simulink model "complex_multiply_example"  (R2023a)
settings: Solver=FixedStepDiscrete  StartTime=0.0  StopTime=100  RelTol=1e-3
PostLoadFcn:
  | % Default delay values
  | D1 = 1;
  | D2 = 1;
  | D3 = 1;
  | D4 = 1;
  | D5 = 1;
InitFcn:
  | % Complex mult input DT
  | InputWL = 18;
  | InputFL = 17;
  | 
  | % Full-precision mult DT
  | MultWL = InputWL*2+1;
  | MultFL = InputFL*2;
  | IntBits = MultWL - MultFL; % integer bits
  | 
  | % Mult DT after rounding
  | OutputWL = 18;
  | OutputFL = OutputWL - IntBits;
settings Model: DataTypeOverride=Off  Creator=cchung  LastModifiedBy=cchung
settings SolverCC: AlgebraicLoopSolver=TrustRegion
settings DataIOCC: LimitDataPoints=on  SaveFormat=Array  SaveOutput=off  SaveTime=off  ReturnWorkspaceOutputs=off
settings OptimizationCC: BlockReduction=off  BooleanDataType=off  ConditionallyExecuteInputs=off  DefaultParameterBehavior=Inlined  LifeSpan=inf
settings DebuggingCC: AlgebraicLoopMsg=error  SaveWithParameterizedLinksMsg=none  UnderspecifiedInitializationDetection=Classic  MergeDetectMultiDrivingBlocksExec=none  SignalResolutionControl=TryResolveAllWithWarning  SingleTaskRateTransMsg=error  UnconnectedInputMsg=warning  UnconnectedOutputMsg=warning  UnconnectedLineMsg=warning  StrictBusMsg=ErrorOnBusTreatedAsVector  SFUnexpectedBacktrackingDiag=warning  SFNoUnconditionalDefaultTransitionDiag=warning  SFExecutionAtInitializationDiag=none  ArithmeticOperatorsInVariantConditions=warning
settings HardwareCC: ProdBitPerPointer=32  ProdBitPerSizeT=32  ProdBitPerPtrDiffT=32  ProdLargestAtomicFloat=None  ProdIntDivRoundTo=Undefined  ProdEndianess=Unspecified  ProdWordSize=32  ProdHWDeviceType=ASIC/FPGA->ASIC/FPGA  TargetUnknown=on  ProdEqTarget=off
settings ModelReferenceCC: EnableRefExpFcnMdlSchedulingChecks=on  PropagateSignalLabelsOutOfModel=off
settings SFSimCC: SimUseLocalCustomCode=off  CustomCodeUndefinedFunction=UseInterfaceOnly
settings RTWCC: RTWUseLocalCustomCode=off
settings CodeAppCC: StateflowObjectComments=on
settings GRTTargetCC: TargetLangStandard=C89/C90 (ANSI)
settings ConfigComp: CovMetricSettings=dw  CovSaveCumulativeToWorkspaceVar=on  CovSaveSingleToWorkspaceVar=on  CovExternalEMLEnable=off

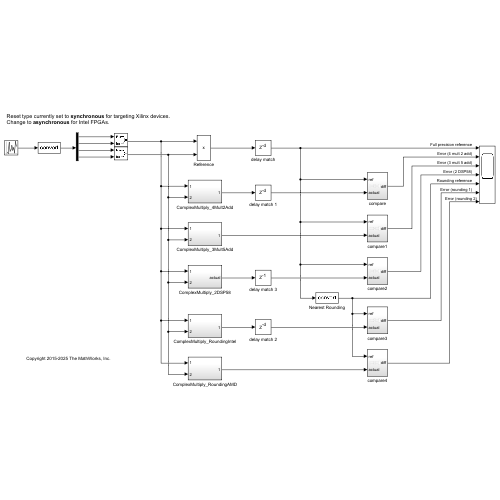
[thumbnail: Simulink's stored preview of the top-level diagram]
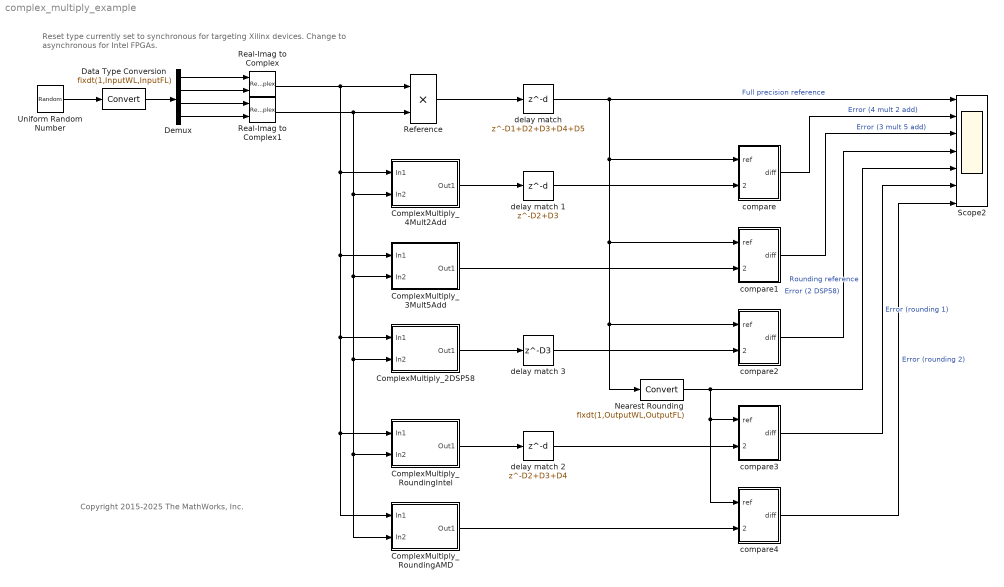
== system complex_multiply_example ==
  note: Copyright 2015-2025 The MathWorks, Inc.
  note: Reset type currently set to synchronous for targeting Xilinx devices.
      | Change to asynchronous for Intel FPGAs.
  ComplexMultiply_2DSP58 : Subsystem
  ComplexMultiply_3Mult5Add : Subsystem
  ComplexMultiply_4Mult2Add : Subsystem
  ComplexMultiply_RoundingAMD : Subsystem
  ComplexMultiply_RoundingIntel : Subsystem
  Data Type Conversion : DataTypeConversion  OutDataTypeStr=fixdt(1,InputWL,InputFL)  RndMeth=Floor
  Demux : Demux
  Nearest Rounding : DataTypeConversion  OutDataTypeStr=fixdt(1,OutputWL,OutputFL)  RndMeth=Nearest  SaturateOnIntegerOverflow=off
  Real-Imag to Complex : RealImagToComplex
  Real-Imag to Complex1 : RealImagToComplex
  Reference : Product  OutDataTypeStr=fixdt(1,MultWL,MultFL)
  Scope2 : Scope  NumInputPorts=7
  Uniform Random Number : UniformRandomNumber  Minimum=-1*ones(1,4)  Maximum=ones(1,4)  Seed=randi([0 100],1,4)  SampleTime=1
  compare : Subsystem
  compare1 : Subsystem
  compare2 : Subsystem
  compare3 : Subsystem
  compare4 : Subsystem
  delay match : Delay  DelayLength=D1+D2+D3+D4+D5
  delay match 1 : Delay  DelayLength=D2+D3
  delay match 2 : Delay  DelayLength=D2+D3+D4
  delay match 3 : Delay  DelayLength=D3
  wires:
  ComplexMultiply_4Mult2Add/1(Out1) -> delay match 1/1
  Real-Imag to Complex/1 -> ComplexMultiply_2DSP58/1(In1), ComplexMultiply_RoundingAMD/1(In1), ComplexMultiply_RoundingIntel/1(In1), ComplexMultiply_3Mult5Add/1(In1), ComplexMultiply_4Mult2Add/1(In1), Reference/1
  Real-Imag to Complex1/1 -> ComplexMultiply_3Mult5Add/2(In2), ComplexMultiply_2DSP58/2(In2), ComplexMultiply_RoundingAMD/2(In2), ComplexMultiply_RoundingIntel/2(In2), ComplexMultiply_4Mult2Add/2(In2), Reference/2
  Reference/1 -> delay match/1
  delay match 1/1 -> compare/2(actual)
  ComplexMultiply_3Mult5Add/1(Out1) -> compare1/2(actual)
  Uniform Random Number/1 -> Data Type Conversion/1
  Data Type Conversion/1 -> Demux/1
  Demux/1 -> Real-Imag to Complex/1
  ComplexMultiply_RoundingIntel/1(Out1) -> delay match 2/1
  delay match/1 -> compare2/1(ref), Nearest Rounding/1, compare1/1(ref), compare/1(ref), Scope2/1  "Full precision reference"
  compare/1(diff) -> Scope2/2  "Error (4 mult 2 add)"
  compare1/1(diff) -> Scope2/3  "Error (3 mult 5 add)"
  delay match 2/1 -> compare3/2(actual)
  Nearest Rounding/1 -> compare4/1(ref), compare3/1(ref), Scope2/5  "Rounding reference"
  Demux/2 -> Real-Imag to Complex/2
  Demux/3 -> Real-Imag to Complex1/1
  Demux/4 -> Real-Imag to Complex1/2
  compare3/1(diff) -> Scope2/6  "Error (rounding 1)"
  ComplexMultiply_RoundingAMD/1(Out1) -> compare4/2(actual)
  compare4/1(diff) -> Scope2/7  "Error (rounding 2)"
  ComplexMultiply_2DSP58/1(Out1) -> delay match 3/1
  delay match 3/1 -> compare2/2(actual)
  compare2/1(diff) -> Scope2/4  "Error (2 DSP58)"

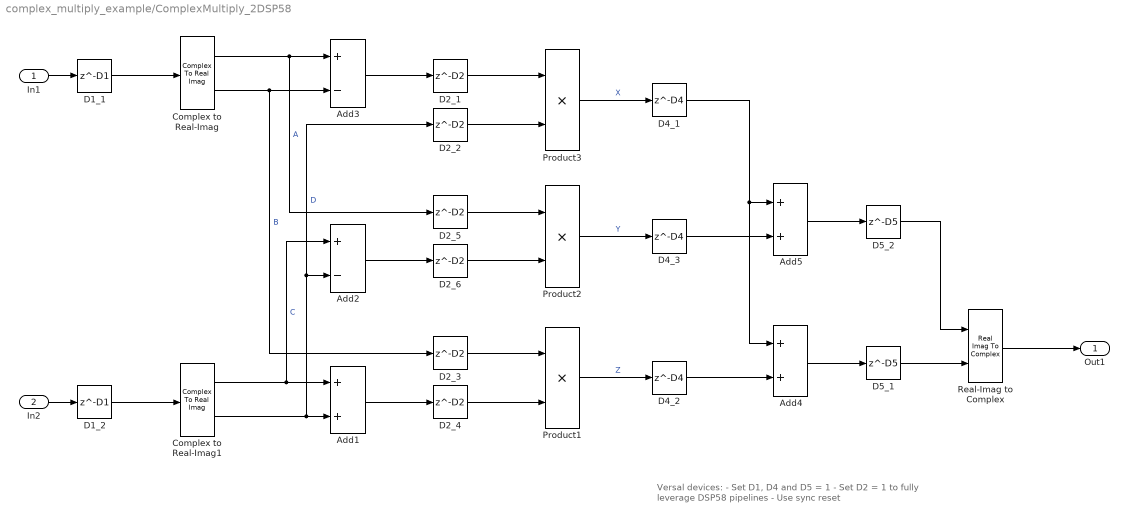
== system complex_multiply_example/ComplexMultiply_2DSP58 ==
  note: Versal devices:
      | - Set D1, D4 and D5 = 1
      | - Set D2 = 1 to fully leverage DSP58 pipelines
      | - Use sync reset
  In1 : Inport
  In2 : Inport  Port=2
  Add1 : Sum
  Add2 : Sum  Inputs=+-
  Add3 : Sum  Inputs=+-
  Add4 : Sum
  Add5 : Sum
  Complex to Real-Imag : ComplexToRealImag
  Complex to Real-Imag1 : ComplexToRealImag
  D1_1 : Delay  DelayLength=D1
  D1_2 : Delay  DelayLength=D1
  D2_{1..6} (6 alike) : Delay  DelayLength=D2
  D4_1 : Delay  DelayLength=D4
  D4_2 : Delay  DelayLength=D4
  D4_3 : Delay  DelayLength=D4
  D5_1 : Delay  DelayLength=D5
  D5_2 : Delay  DelayLength=D5
  Product1 : Product
  Product2 : Product
  Product3 : Product
  Real-Imag to Complex : RealImagToComplex
  Out1 : Outport  VectorParamsAs1DForOutWhenUnconnected=off
  wires:
  Real-Imag to Complex/1 -> Out1/1
  In2/1 -> D1_2/1
  Complex to Real-Imag1/1 -> Add2/1, Add1/1  "C"
  Add4/1 -> D5_1/1
  Add5/1 -> D5_2/1
  In1/1 -> D1_1/1
  D1_1/1 -> Complex to Real-Imag/1
  D1_2/1 -> Complex to Real-Imag1/1
  Complex to Real-Imag/1 -> Add3/1, D2_5/1  "A"
  Complex to Real-Imag/2 -> Add3/2, D2_3/1  "B"
  Add3/1 -> D2_1/1
  Complex to Real-Imag1/2 -> D2_2/1, Add2/2, Add1/2  "D"
  Add1/1 -> D2_4/1
  Add2/1 -> D2_6/1
  Product3/1 -> D4_1/1  "X"
  Product1/1 -> D4_2/1  "Z"
  Product2/1 -> D4_3/1  "Y"
  D5_1/1 -> Real-Imag to Complex/2
  D5_2/1 -> Real-Imag to Complex/1
  D4_1/1 -> Add4/1, Add5/1
  D4_2/1 -> Add4/2
  D4_3/1 -> Add5/2
  D2_1/1 -> Product3/1
  D2_2/1 -> Product3/2
  D2_3/1 -> Product1/1
  D2_4/1 -> Product1/2
  D2_5/1 -> Product2/1
  D2_6/1 -> Product2/2

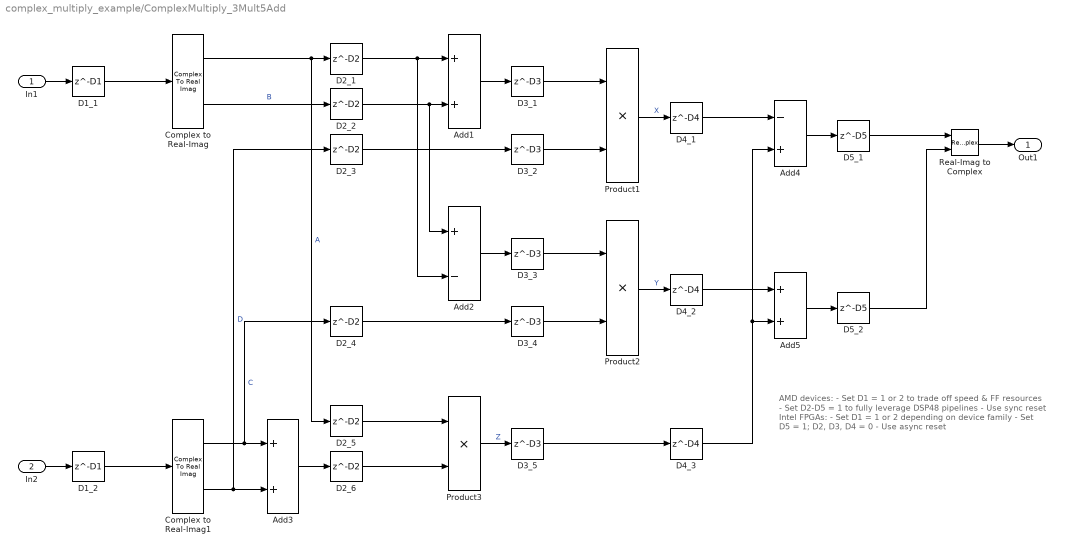
== system complex_multiply_example/ComplexMultiply_3Mult5Add ==
  note: AMD devices:
      | - Set D1 = 1 or 2 to trade off speed & FF resources
      | - Set D2-D5 = 1 to fully leverage DSP48 pipelines
      | - Use sync reset
      |
      | Intel FPGAs:
      | - Set D1 = 1 or 2 depending on device family
      | - Set D5 = 1; D2, D3, D4 = 0
      | - Use async reset
  In1 : Inport
  In2 : Inport  Port=2
  Add1 : Sum
  Add2 : Sum  Inputs=+-
  Add3 : Sum
  Add4 : Sum  Inputs=-+
  Add5 : Sum
  Complex to Real-Imag : ComplexToRealImag
  Complex to Real-Imag1 : ComplexToRealImag
  D1_1 : Delay  DelayLength=D1
  D1_2 : Delay  DelayLength=D1
  D2_{1..6} (6 alike) : Delay  DelayLength=D2
  D3_{1..5} (5 alike) : Delay  DelayLength=D3
  D4_1 : Delay  DelayLength=D4
  D4_2 : Delay  DelayLength=D4
  D4_3 : Delay  DelayLength=D4
  D5_1 : Delay  DelayLength=D5
  D5_2 : Delay  DelayLength=D5
  Product1 : Product
  Product2 : Product
  Product3 : Product
  Real-Imag to Complex : RealImagToComplex
  Out1 : Outport  VectorParamsAs1DForOutWhenUnconnected=off
  wires:
  Real-Imag to Complex/1 -> Out1/1
  In2/1 -> D1_2/1
  Complex to Real-Imag1/1 -> Add3/1, D2_4/1  "C"
  Complex to Real-Imag1/2 -> Add3/2, D2_3/1  "D"
  Product1/1 -> D4_1/1  "X"
  Product2/1 -> D4_2/1  "Y"
  Product3/1 -> D3_5/1  "Z"
  Add4/1 -> D5_1/1
  Add5/1 -> D5_2/1
  D5_1/1 -> Real-Imag to Complex/1
  D5_2/1 -> Real-Imag to Complex/2
  D4_1/1 -> Add4/1
  D4_2/1 -> Add5/1
  D3_5/1 -> D4_3/1
  Add1/1 -> D3_1/1
  Add3/1 -> D2_6/1
  Add2/1 -> D3_3/1
  Complex to Real-Imag/1 -> D2_5/1, D2_1/1  "A"
  Complex to Real-Imag/2 -> D2_2/1  "B"
  D3_1/1 -> Product1/1
  D2_6/1 -> Product3/2
  D3_3/1 -> Product2/1
  D4_3/1 -> Add4/2, Add5/2
  D3_4/1 -> Product2/2
  D3_2/1 -> Product1/2
  D2_4/1 -> D3_4/1
  D2_3/1 -> D3_2/1
  D2_5/1 -> Product3/1
  D2_2/1 -> Add1/2, Add2/1
  D2_1/1 -> Add2/2, Add1/1
  In1/1 -> D1_1/1
  D1_1/1 -> Complex to Real-Imag/1
  D1_2/1 -> Complex to Real-Imag1/1

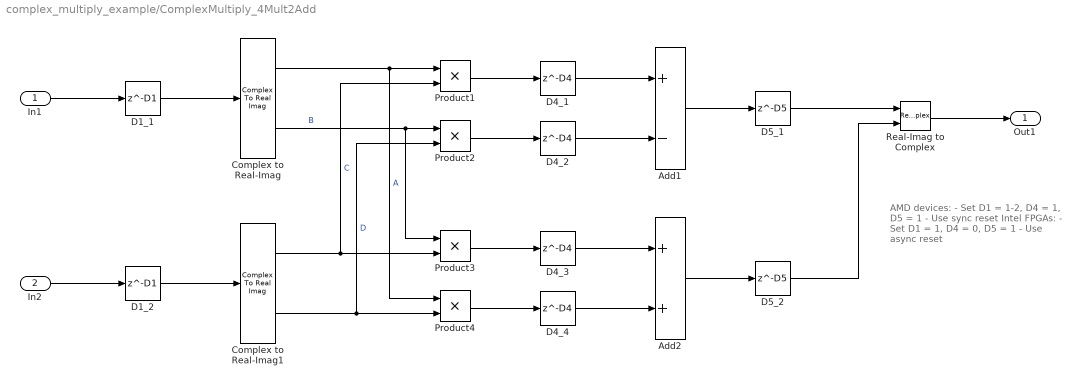
== system complex_multiply_example/ComplexMultiply_4Mult2Add ==
  note: AMD devices:
      | - Set D1 = 1-2, D4 = 1, D5 = 1
      | - Use sync reset
      |
      | Intel FPGAs:
      | - Set D1 = 1, D4 = 0, D5 = 1
      | - Use async reset
  In1 : Inport
  In2 : Inport  Port=2
  Add1 : Sum  Inputs=+-
  Add2 : Sum
  Complex to Real-Imag : ComplexToRealImag
  Complex to Real-Imag1 : ComplexToRealImag
  D1_1 : Delay  DelayLength=D1
  D1_2 : Delay  DelayLength=D1
  D4_{1..4} (4 alike) : Delay  DelayLength=D4
  D5_1 : Delay  DelayLength=D5
  D5_2 : Delay  DelayLength=D5
  Product{1..4} (4 alike) : Product
  Real-Imag to Complex : RealImagToComplex
  Out1 : Outport  VectorParamsAs1DForOutWhenUnconnected=off
  wires:
  In2/1 -> D1_2/1
  In1/1 -> D1_1/1
  Real-Imag to Complex/1 -> Out1/1
  D1_1/1 -> Complex to Real-Imag/1
  D1_2/1 -> Complex to Real-Imag1/1
  Complex to Real-Imag/1 -> Product4/1, Product1/1  "A"
  Complex to Real-Imag1/1 -> Product3/2, Product1/2  "C"
  Complex to Real-Imag/2 -> Product3/1, Product2/1  "B"
  Complex to Real-Imag1/2 -> Product4/2, Product2/2  "D"
  Product1/1 -> D4_1/1
  Product3/1 -> D4_3/1
  Add1/1 -> D5_1/1
  Add2/1 -> D5_2/1
  D5_1/1 -> Real-Imag to Complex/1
  D5_2/1 -> Real-Imag to Complex/2
  D4_1/1 -> Add1/1
  Product2/1 -> D4_2/1
  D4_3/1 -> Add2/1
  Product4/1 -> D4_4/1
  D4_2/1 -> Add1/2
  D4_4/1 -> Add2/2

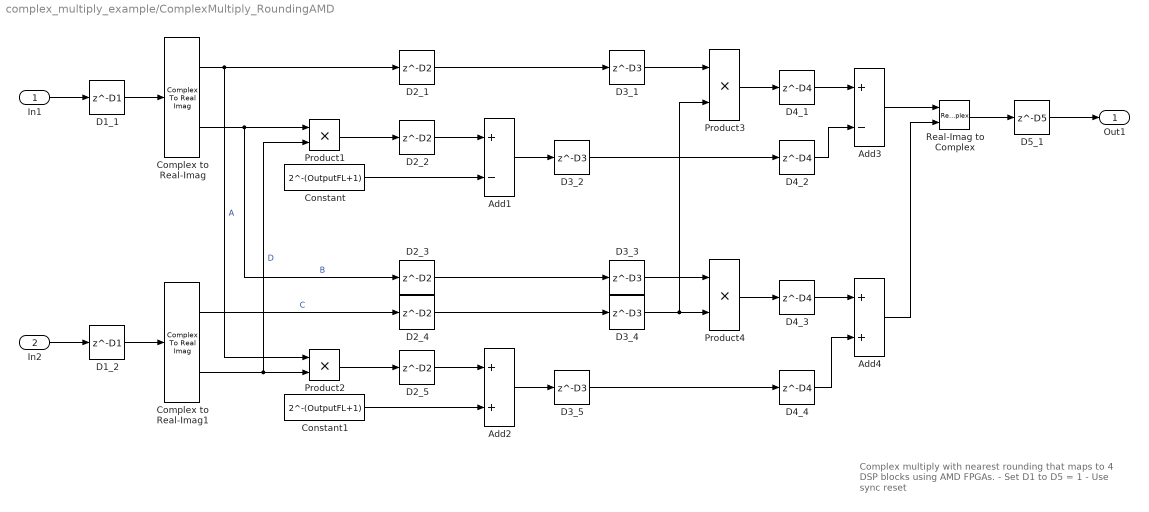
== system complex_multiply_example/ComplexMultiply_RoundingAMD ==
  note: Complex multiply with nearest rounding that maps to 4 DSP blocks using AMD FPGAs.
      |
      | - Set D1 to D5 = 1
      | - Use sync reset
  In1 : Inport
  In2 : Inport  Port=2
  Add1 : Sum  Inputs=+-
  Add2 : Sum
  Add3 : Sum  Inputs=+-  OutDataTypeStr=fixdt(1,OutputWL,OutputFL)
  Add4 : Sum  OutDataTypeStr=fixdt(1,OutputWL,OutputFL)
  Complex to Real-Imag : ComplexToRealImag
  Complex to Real-Imag1 : ComplexToRealImag
  Constant : Constant  Value=2^-(OutputFL+1)  OutDataTypeStr=Inherit: Inherit via back propagation  SampleTime=-1
  Constant1 : Constant  Value=2^-(OutputFL+1)  OutDataTypeStr=Inherit: Inherit via back propagation  SampleTime=-1
  D1_1 : Delay  DelayLength=D1
  D1_2 : Delay  DelayLength=D1
  D2_{1..5} (5 alike) : Delay  DelayLength=D2
  D3_{1..5} (5 alike) : Delay  DelayLength=D3
  D4_{1..4} (4 alike) : Delay  DelayLength=D4
  D5_1 : Delay  DelayLength=D5
  Product{1..4} (4 alike) : Product
  Real-Imag to Complex : RealImagToComplex
  Out1 : Outport  VectorParamsAs1DForOutWhenUnconnected=off
  wires:
  In2/1 -> D1_2/1
  In1/1 -> D1_1/1
  D1_1/1 -> Complex to Real-Imag/1
  D1_2/1 -> Complex to Real-Imag1/1
  Complex to Real-Imag/1 -> D2_1/1, Product2/1  "A"
  Complex to Real-Imag1/1 -> D2_4/1  "C"
  Complex to Real-Imag/2 -> Product1/1, D2_3/1  "B"
  Complex to Real-Imag1/2 -> Product2/2, Product1/2  "D"
  Product1/1 -> D2_2/1
  Real-Imag to Complex/1 -> D5_1/1
  Add1/1 -> D3_2/1
  Add4/1 -> Real-Imag to Complex/2
  D5_1/1 -> Out1/1
  Add3/1 -> Real-Imag to Complex/1
  Constant/1 -> Add1/2
  Product3/1 -> D4_1/1
  Product2/1 -> D2_5/1
  Constant1/1 -> Add2/2
  Add2/1 -> D3_5/1
  Product4/1 -> D4_3/1
  D3_5/1 -> D4_4/1
  D3_1/1 -> Product3/1
  D3_2/1 -> D4_2/1
  D3_3/1 -> Product4/1
  D3_4/1 -> Product3/2, Product4/2
  D4_1/1 -> Add3/1
  D4_2/1 -> Add3/2
  D4_3/1 -> Add4/1
  D4_4/1 -> Add4/2
  D2_1/1 -> D3_1/1
  D2_2/1 -> Add1/1
  D2_3/1 -> D3_3/1
  D2_4/1 -> D3_4/1
  D2_5/1 -> Add2/1

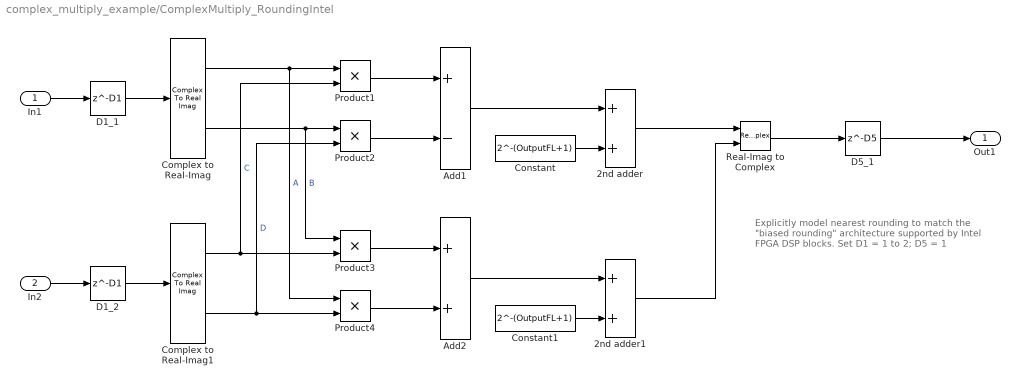
== system complex_multiply_example/ComplexMultiply_RoundingIntel ==
  note: Explicitly model nearest rounding to match the "biased rounding" architecture supported by Intel FPGA DSP blocks.
      |
      | Set D1 = 1 to 2; D5 = 1
  In1 : Inport
  In2 : Inport  Port=2
  2nd adder : Sum  OutDataTypeStr=fixdt(1,OutputWL,OutputFL)
  2nd adder1 : Sum  OutDataTypeStr=fixdt(1,OutputWL,OutputFL)
  Add1 : Sum  Inputs=+-
  Add2 : Sum
  Complex to Real-Imag : ComplexToRealImag
  Complex to Real-Imag1 : ComplexToRealImag
  Constant : Constant  Value=2^-(OutputFL+1)  OutDataTypeStr=Inherit: Inherit via back propagation  SampleTime=-1
  Constant1 : Constant  Value=2^-(OutputFL+1)  OutDataTypeStr=Inherit: Inherit via back propagation  SampleTime=-1
  D1_1 : Delay  DelayLength=D1
      settings: AttributesFormatString=ResetType : none
  D1_2 : Delay  DelayLength=D1
      settings: AttributesFormatString=ResetType : none
  D5_1 : Delay  DelayLength=D5
      settings: AttributesFormatString=ResetType : none
  Product{1..4} (4 alike) : Product
  Real-Imag to Complex : RealImagToComplex
  Out1 : Outport  VectorParamsAs1DForOutWhenUnconnected=off
  wires:
  In2/1 -> D1_2/1
  In1/1 -> D1_1/1
  D1_1/1 -> Complex to Real-Imag/1
  D1_2/1 -> Complex to Real-Imag1/1
  Complex to Real-Imag/1 -> Product4/1, Product1/1  "A"
  Complex to Real-Imag1/1 -> Product3/2, Product1/2  "C"
  Complex to Real-Imag/2 -> Product3/1, Product2/1  "B"
  Complex to Real-Imag1/2 -> Product4/2, Product2/2  "D"
  Product1/1 -> Add1/1
  Product3/1 -> Add2/1
  Product2/1 -> Add1/2
  Product4/1 -> Add2/2
  Real-Imag to Complex/1 -> D5_1/1
  Add1/1 -> 2nd adder/1
  2nd adder1/1 -> Real-Imag to Complex/2
  Add2/1 -> 2nd adder1/1
  D5_1/1 -> Out1/1
  Constant/1 -> 2nd adder/2
  Constant1/1 -> 2nd adder1/2
  2nd adder/1 -> Real-Imag to Complex/1

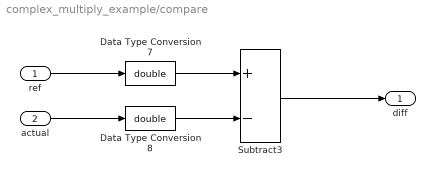
== system complex_multiply_example/compare ==
  ref : Inport
  actual : Inport  Port=2
  Data Type Conversion7 : DataTypeConversion  OutDataTypeStr=double  SaturateOnIntegerOverflow=off  RndMeth=Floor
  Data Type Conversion8 : DataTypeConversion  OutDataTypeStr=double  SaturateOnIntegerOverflow=off  RndMeth=Floor
  Subtract3 : Sum  Inputs=+-
  diff : Outport  VectorParamsAs1DForOutWhenUnconnected=off
  wires:
  actual/1 -> Data Type Conversion8/1
  Data Type Conversion7/1 -> Subtract3/1
  Data Type Conversion8/1 -> Subtract3/2
  ref/1 -> Data Type Conversion7/1
  Subtract3/1 -> diff/1

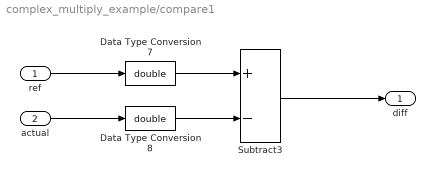
== system complex_multiply_example/compare1 ==
  ref : Inport
  actual : Inport  Port=2
  Data Type Conversion7 : DataTypeConversion  OutDataTypeStr=double  SaturateOnIntegerOverflow=off  RndMeth=Floor
  Data Type Conversion8 : DataTypeConversion  OutDataTypeStr=double  SaturateOnIntegerOverflow=off  RndMeth=Floor
  Subtract3 : Sum  Inputs=+-
  diff : Outport  VectorParamsAs1DForOutWhenUnconnected=off
  wires:
  actual/1 -> Data Type Conversion8/1
  Data Type Conversion7/1 -> Subtract3/1
  Data Type Conversion8/1 -> Subtract3/2
  ref/1 -> Data Type Conversion7/1
  Subtract3/1 -> diff/1

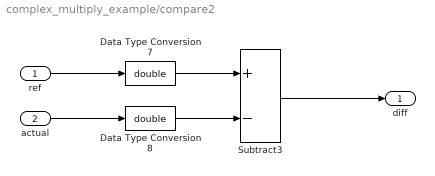
== system complex_multiply_example/compare2 ==
  ref : Inport
  actual : Inport  Port=2
  Data Type Conversion7 : DataTypeConversion  OutDataTypeStr=double  SaturateOnIntegerOverflow=off  RndMeth=Floor
  Data Type Conversion8 : DataTypeConversion  OutDataTypeStr=double  SaturateOnIntegerOverflow=off  RndMeth=Floor
  Subtract3 : Sum  Inputs=+-
  diff : Outport  VectorParamsAs1DForOutWhenUnconnected=off
  wires:
  actual/1 -> Data Type Conversion8/1
  Data Type Conversion7/1 -> Subtract3/1
  Data Type Conversion8/1 -> Subtract3/2
  ref/1 -> Data Type Conversion7/1
  Subtract3/1 -> diff/1

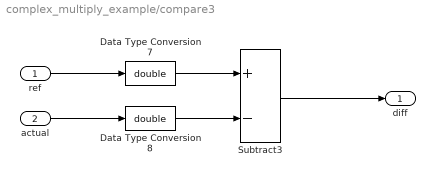
== system complex_multiply_example/compare3 ==
  ref : Inport
  actual : Inport  Port=2
  Data Type Conversion7 : DataTypeConversion  OutDataTypeStr=double  SaturateOnIntegerOverflow=off  RndMeth=Floor
  Data Type Conversion8 : DataTypeConversion  OutDataTypeStr=double  SaturateOnIntegerOverflow=off  RndMeth=Floor
  Subtract3 : Sum  Inputs=+-
  diff : Outport  VectorParamsAs1DForOutWhenUnconnected=off
  wires:
  actual/1 -> Data Type Conversion8/1
  Data Type Conversion7/1 -> Subtract3/1
  Data Type Conversion8/1 -> Subtract3/2
  ref/1 -> Data Type Conversion7/1
  Subtract3/1 -> diff/1

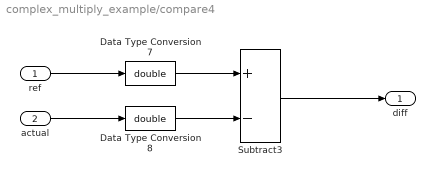
== system complex_multiply_example/compare4 ==
  ref : Inport
  actual : Inport  Port=2
  Data Type Conversion7 : DataTypeConversion  OutDataTypeStr=double  SaturateOnIntegerOverflow=off  RndMeth=Floor
  Data Type Conversion8 : DataTypeConversion  OutDataTypeStr=double  SaturateOnIntegerOverflow=off  RndMeth=Floor
  Subtract3 : Sum  Inputs=+-
  diff : Outport  VectorParamsAs1DForOutWhenUnconnected=off
  wires:
  actual/1 -> Data Type Conversion8/1
  Data Type Conversion7/1 -> Subtract3/1
  Data Type Conversion8/1 -> Subtract3/2
  ref/1 -> Data Type Conversion7/1
  Subtract3/1 -> diff/1
